simulink library "WECSim_Lib"  (R2015b)
settings: Solver=ode45  StartTime=0.0  StopTime=10.0  RelTol=1e-3
undefined symbols (not defined in the file): body, constraint, mooring, pto, simu, waves, X, Y, Z
libraries: nesl_utility x168, sm_lib x94, vrlib x12
(part 6 of 7)

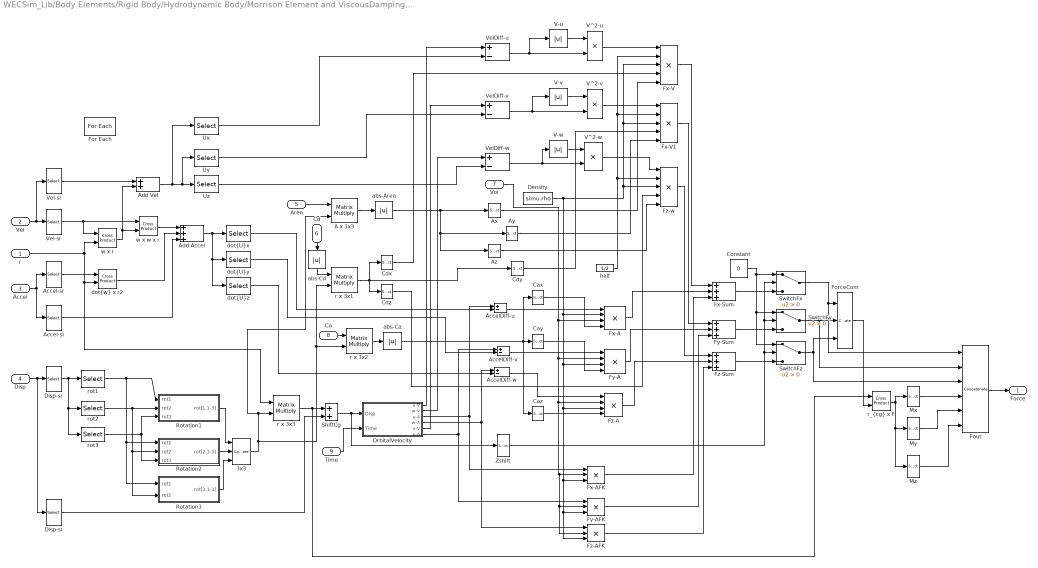
== system WECSim_Lib/Body Elements/Rigid Body/Hydrodynamic Body/Morrison Element and ViscousDampingForceCalculation/Morrison Element Variant Subsystem/Morrison Element On/No Wave Excitation Force/MorrisonElements ==
  r : Inport  Partition=on  PartitionDimension=1  PartitionWidth=1
  Vel : Inport  Port=2
  Accel : Inport  Port=3
  Disp : Inport  Port=4
  Area : Inport  Port=5  Partition=on  PartitionDimension=1  PartitionWidth=1
  Cd : Inport  Port=6  Partition=on  PartitionDimension=1  PartitionWidth=1
  Vol : Inport  Port=7  Partition=on  PartitionDimension=1  PartitionWidth=1
  Ca : Inport  Port=8  Partition=on  PartitionDimension=1  PartitionWidth=1
  Time : Inport  Port=9
  3x3 : Concatenate  NumInputs=3  Mode=Multidimensional array
  A x 3x3 : Product  Multiplication=Matrix(*)
  Accel-sl : Selector  InputPortWidth=6  IndexOptions=Index vector (dialog)  Indices=[1 2 3]  OutputSizes=1
  Accel-sr : Selector  InputPortWidth=6  IndexOptions=Index vector (dialog)  Indices=[4 5 6]  OutputSizes=1
  AccelDiff-u : Sum  Inputs=+-
  AccelDiff-v : Sum  Inputs=+-
  AccelDiff-w : Sum  Inputs=+-
  Add Accel : Sum  Inputs=+++
  Add Vel : Sum
  Ax : Selector  InputPortWidth=3  IndexOptions=Index vector (dialog)  Indices=[1]  OutputSizes=1
  Ay : Selector  InputPortWidth=3  IndexOptions=Index vector (dialog)  Indices=[2]  OutputSizes=1
  Az : Selector  InputPortWidth=3  IndexOptions=Index vector (dialog)  Indices=[3]  OutputSizes=1
  Cax : Selector  InputPortWidth=3  IndexOptions=Index vector (dialog)  Indices=[1]  OutputSizes=1
  Cay : Selector  InputPortWidth=3  IndexOptions=Index vector (dialog)  Indices=[2]  OutputSizes=1
  Caz : Selector  InputPortWidth=3  IndexOptions=Index vector (dialog)  Indices=[3]  OutputSizes=1
  Cdx : Selector  InputPortWidth=3  IndexOptions=Index vector (dialog)  Indices=[1]  OutputSizes=1
  Cdy : Selector  InputPortWidth=3  IndexOptions=Index vector (dialog)  Indices=[2]  OutputSizes=1
  Cdz : Selector  InputPortWidth=3  IndexOptions=Index vector (dialog)  Indices=[3]  OutputSizes=1
  Constant : Constant  Value=0
  Density : Constant  Value=simu.rho
  Disp-sl : Selector  InputPortWidth=6  IndexOptions=Index vector (dialog)  Indices=[1 2 3]  OutputSizes=1
  Disp-sr : Selector  InputPortWidth=6  IndexOptions=Index vector (dialog)  Indices=[4 5 6]  OutputSizes=1
  For Each : ForEach  DisableCoverage=on  IndexMode=One-based
  ForceCom : Concatenate  NumInputs=3  ConcatenateDimension=2
  Fout : Concatenate  NumInputs=6  Mode=Multidimensional array  ConcatenateDimension=2
  Fx-A : Product  Inputs=4
  Fx-AFK : Product  Inputs=3
  Fx-Sum : Sum  Inputs=+++
  Fx-V : Product  Inputs=5
  Fx-V1 : Product  Inputs=5
  Fy-A : Product  Inputs=4
  Fy-AFK : Product  Inputs=3
  Fy-Sum : Sum  Inputs=+++
  Fz-A : Product  Inputs=4
  Fz-AFK : Product  Inputs=3
  Fz-Sum : Sum  Inputs=+++
  Fz-w : Product  Inputs=5
  Mx : Selector  InputPortWidth=3  IndexOptions=Index vector (dialog)  Indices=[1]  OutputSizes=1
  My : Selector  InputPortWidth=3  IndexOptions=Index vector (dialog)  Indices=[2]  OutputSizes=1
  Mz : Selector  InputPortWidth=3  IndexOptions=Index vector (dialog)  Indices=[3]  OutputSizes=1
  OrbitalVelocity : Subsystem
  Rotation1 : Subsystem
  Rotation2 : Subsystem
  Rotation3 : Subsystem
  ShiftCg : Sum
  SwitchFx : Switch  Criteria=u2 > Threshold
  SwitchFy : Switch  Criteria=u2 > Threshold
  SwitchFz : Switch  Criteria=u2 > Threshold
  Ux : Selector  InputPortWidth=3  IndexOptions=Index vector (dialog)  Indices=[1]  OutputSizes=1
  Uy : Selector  InputPortWidth=3  IndexOptions=Index vector (dialog)  Indices=[2]  OutputSizes=1
  Uz : Selector  InputPortWidth=3  IndexOptions=Index vector (dialog)  Indices=[3]  OutputSizes=1
  V-u : Abs
  V-v : Abs
  V-w : Abs
  V^2-u : Product
  V^2-v : Product
  V^2-w : Product
  Vel-sl : Selector  InputPortWidth=6  IndexOptions=Index vector (dialog)  Indices=[1 2 3]  OutputSizes=1
  "Vel-sr " : Selector  InputPortWidth=6  IndexOptions=Index vector (dialog)  Indices=[4 5 6]  OutputSizes=1
  VelDiff-u : Sum  Inputs=+-
  VelDiff-v : Sum  Inputs=+-
  VelDiff-w : Sum  Inputs=+-
  Zshift : Selector  InputPortWidth=3  IndexOptions=Index vector (dialog)  Indices=[3]  OutputSizes=1
  abs-Area : Abs
  abs-Ca : Abs
  abs-Cd : Abs
  "dot{U}x" : Selector  InputPortWidth=3  IndexOptions=Index vector (dialog)  Indices=[1]  OutputSizes=1
  "dot{U}y" : Selector  InputPortWidth=3  IndexOptions=Index vector (dialog)  Indices=[2]  OutputSizes=1
  "dot{U}z" : Selector  InputPortWidth=3  IndexOptions=Index vector (dialog)  Indices=[3]  OutputSizes=1
  "dot{w} x r2" : vrlib/Utilities/Cross Product
  half : Constant  Value=1/2
  r x 3x1 : Product  Multiplication=Matrix(*)
  r x 3x2 : Product  Multiplication=Matrix(*)
  r x 3x3 : Product  Multiplication=Matrix(*)
  "r_{cg} x F" : vrlib/Utilities/Cross Product
  rot1 : Selector  InputPortWidth=3  IndexOptions=Index vector (dialog)  Indices=[1]  OutputSizes=1
  rot2 : Selector  InputPortWidth=3  IndexOptions=Index vector (dialog)  Indices=[2]  OutputSizes=1
  rot3 : Selector  InputPortWidth=3  IndexOptions=Index vector (dialog)  Indices=[3]  OutputSizes=1
  w x r : vrlib/Utilities/Cross Product
  w x w x r : vrlib/Utilities/Cross Product
  Force : Outport  PortDimensions=[1 6]  ConcatenationDimension=1
  wires:
  Vel/1 -> Vel-sl/1, "Vel-sr "/1
  w x r/1 -> Add Vel/2, w x w x r/2
  w x w x r/1 -> Add Accel/1
  "Vel-sr "/1 -> w x w x r/1, w x r/1
  r/1 -> r x 3x3/1, "dot{w} x r2"/2, w x r/2
  Accel/1 -> Accel-sl/1, Accel-sr/1
  Accel-sr/1 -> "dot{w} x r2"/1
  "dot{w} x r2"/1 -> Add Accel/2
  Accel-sl/1 -> Add Accel/3
  Add Accel/1 -> "dot{U}z"/1, "dot{U}y"/1, "dot{U}x"/1
  Vel-sl/1 -> Add Vel/1
  Disp/1 -> Disp-sl/1, Disp-sr/1
  Disp-sr/1 -> rot3/1, rot2/1, rot1/1
  rot3/1 -> Rotation2/3(rot3), Rotation1/3(rot3)
  rot1/1 -> Rotation3/1(rot1), Rotation2/1(rot1), Rotation1/1(rot1)
  rot2/1 -> Rotation3/2(rot2), Rotation2/2(rot2), Rotation1/2(rot2)
  Rotation2/1(rot[2,1-3]) -> 3x3/2
  Rotation1/1(rot[1,1-3]) -> 3x3/1
  Rotation3/1(rot[3,1-3]) -> 3x3/3
  r x 3x3/1 -> "r_{cg} x F"/1, ShiftCg/1
  Disp-sl/1 -> ShiftCg/2
  ShiftCg/1 -> Zshift/1, OrbitalVelocity/1(Disp)
  "dot{U}y"/1 -> AccelDiff-v/2
  "dot{U}x"/1 -> AccelDiff-u/2
  OrbitalVelocity/3(u-A) -> AccelDiff-u/1, Fx-AFK/1
  "dot{U}z"/1 -> AccelDiff-w/2
  Add Vel/1 -> Uy/1, Uz/1, Ux/1
  Uy/1 -> VelDiff-v/2
  Ux/1 -> VelDiff-u/2
  Uz/1 -> VelDiff-w/2
  OrbitalVelocity/1(u-V) -> VelDiff-u/1
  OrbitalVelocity/2(w-V) -> VelDiff-w/1
  VelDiff-w/1 -> V-w/1, V^2-w/2
  V^2-u/1 -> Fx-V/1
  half/1 -> Fz-w/2, Fx-V1/2, Fx-V/2
  Density/1 -> Fy-A/3, Fy-AFK/3, Fz-AFK/3, Fx-AFK/3, Fz-A/3, Fx-A/2, Fz-w/3, Fx-V1/3, Fx-V/3
  V^2-w/1 -> Fz-w/1
  AccelDiff-u/1 -> Fx-A/1
  Vol/1 -> Fy-A/2, Fy-AFK/2, Fz-AFK/2, Fx-AFK/2, Fz-A/2, Fx-A/3
  AccelDiff-w/1 -> Fz-A/1
  OrbitalVelocity/4(w-A) -> Fz-AFK/1, AccelDiff-w/1
  Fx-V/1 -> Fx-Sum/1
  Fx-A/1 -> Fx-Sum/2
  Fx-AFK/1 -> Fx-Sum/3
  Fz-w/1 -> Fz-Sum/1
  Fz-A/1 -> Fz-Sum/2
  Fz-AFK/1 -> Fz-Sum/3
  "r_{cg} x F"/1 -> Mz/1, My/1, Mx/1
  Mx/1 -> Fout/4
  My/1 -> Fout/5
  Mz/1 -> Fout/6
  3x3/1 -> A x 3x3/2, r x 3x3/2, r x 3x2/2, r x 3x1/2
  V-u/1 -> V^2-u/1
  VelDiff-u/1 -> V-u/1, V^2-u/2
  Zshift/1 -> SwitchFy/2, SwitchFx/2, SwitchFz/2
  SwitchFz/1 -> ForceCom/3, Fout/3
  SwitchFx/1 -> Fout/1, ForceCom/1
  Fx-Sum/1 -> SwitchFx/3
  Fz-Sum/1 -> SwitchFz/3
  Az/1 -> Fz-w/5
  Area/1 -> A x 3x3/1
  Ax/1 -> Fx-V/5
  Cdx/1 -> Fx-V/4
  Cdz/1 -> Fz-w/4
  A x 3x3/1 -> abs-Area/1
  abs-Area/1 -> Ay/1, Az/1, Ax/1
  ForceCom/1 -> "r_{cg} x F"/2
  Fout/1 -> Force/1
  Caz/1 -> Fz-A/4
  Cax/1 -> Fx-A/4
  Cd/1 -> abs-Cd/1
  r x 3x1/1 -> Cdy/1, Cdz/1, Cdx/1
  Ca/1 -> r x 3x2/1
  r x 3x2/1 -> abs-Ca/1
  OrbitalVelocity/6(v-A) -> AccelDiff-v/1, Fy-AFK/1
  V^2-v/1 -> Fx-V1/1
  V-v/1 -> V^2-v/1
  VelDiff-v/1 -> V-v/1, V^2-v/2
  OrbitalVelocity/5(v-V) -> VelDiff-v/1
  Ay/1 -> Fx-V1/5
  Cdy/1 -> Fx-V1/4
  SwitchFy/1 -> Fout/2, ForceCom/2
  Fy-Sum/1 -> SwitchFy/3
  Fy-AFK/1 -> Fy-Sum/3
  AccelDiff-v/1 -> Fy-A/1
  Cay/1 -> Fy-A/4
  Fy-A/1 -> Fy-Sum/2
  Fx-V1/1 -> Fy-Sum/1
  Constant/1 -> SwitchFy/1, SwitchFz/1, SwitchFx/1
  V-w/1 -> V^2-w/1
  abs-Ca/1 -> Cax/1, Cay/1, Caz/1
  abs-Cd/1 -> r x 3x1/1
  Time/1 -> OrbitalVelocity/2(Time)

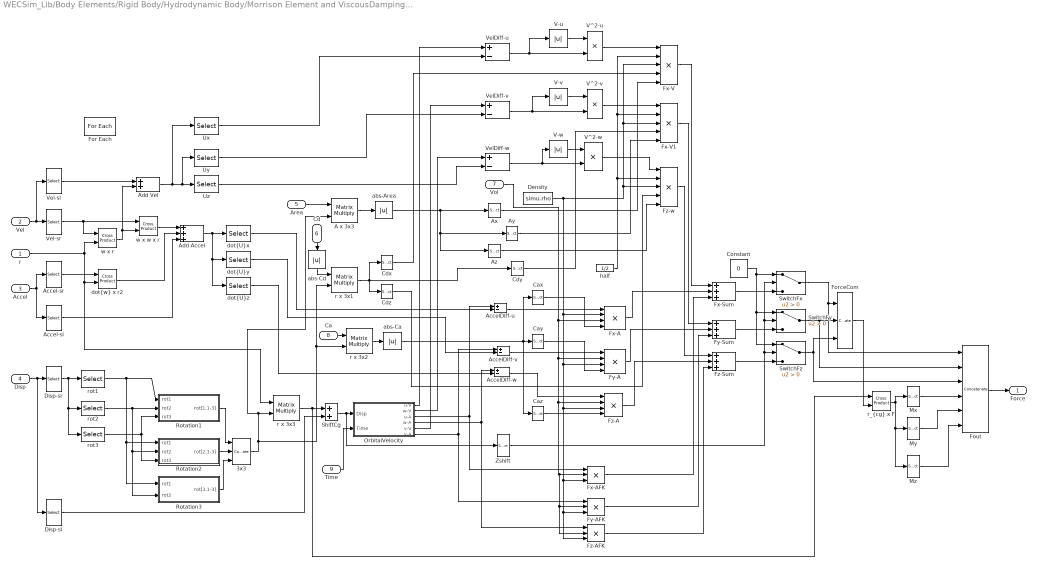
== system WECSim_Lib/Body Elements/Rigid Body/Hydrodynamic Body/Morrison Element and ViscousDampingForceCalculation/Morrison Element Variant Subsystem/Morrison Element On/Regular Wave Excitation Force/MorrisonElements ==
  r : Inport  Partition=on  PartitionDimension=1  PartitionWidth=1
  Vel : Inport  Port=2
  Accel : Inport  Port=3
  Disp : Inport  Port=4
  Area : Inport  Port=5  Partition=on  PartitionDimension=1  PartitionWidth=1
  Cd : Inport  Port=6  Partition=on  PartitionDimension=1  PartitionWidth=1
  Vol : Inport  Port=7  Partition=on  PartitionDimension=1  PartitionWidth=1
  Ca : Inport  Port=8  Partition=on  PartitionDimension=1  PartitionWidth=1
  Time : Inport  Port=9
  3x3 : Concatenate  NumInputs=3  Mode=Multidimensional array
  A x 3x3 : Product  Multiplication=Matrix(*)
  Accel-sl : Selector  InputPortWidth=6  IndexOptions=Index vector (dialog)  Indices=[1 2 3]  OutputSizes=1
  Accel-sr : Selector  InputPortWidth=6  IndexOptions=Index vector (dialog)  Indices=[4 5 6]  OutputSizes=1
  AccelDiff-u : Sum  Inputs=+-
  AccelDiff-v : Sum  Inputs=+-
  AccelDiff-w : Sum  Inputs=+-
  Add Accel : Sum  Inputs=+++
  Add Vel : Sum
  Ax : Selector  InputPortWidth=3  IndexOptions=Index vector (dialog)  Indices=[1]  OutputSizes=1
  Ay : Selector  InputPortWidth=3  IndexOptions=Index vector (dialog)  Indices=[2]  OutputSizes=1
  Az : Selector  InputPortWidth=3  IndexOptions=Index vector (dialog)  Indices=[3]  OutputSizes=1
  Cax : Selector  InputPortWidth=3  IndexOptions=Index vector (dialog)  Indices=[1]  OutputSizes=1
  Cay : Selector  InputPortWidth=3  IndexOptions=Index vector (dialog)  Indices=[2]  OutputSizes=1
  Caz : Selector  InputPortWidth=3  IndexOptions=Index vector (dialog)  Indices=[3]  OutputSizes=1
  Cdx : Selector  InputPortWidth=3  IndexOptions=Index vector (dialog)  Indices=[1]  OutputSizes=1
  Cdy : Selector  InputPortWidth=3  IndexOptions=Index vector (dialog)  Indices=[2]  OutputSizes=1
  Cdz : Selector  InputPortWidth=3  IndexOptions=Index vector (dialog)  Indices=[3]  OutputSizes=1
  Constant : Constant  Value=0
  Density : Constant  Value=simu.rho
  Disp-sl : Selector  InputPortWidth=6  IndexOptions=Index vector (dialog)  Indices=[1 2 3]  OutputSizes=1
  Disp-sr : Selector  InputPortWidth=6  IndexOptions=Index vector (dialog)  Indices=[4 5 6]  OutputSizes=1
  For Each : ForEach  DisableCoverage=on  IndexMode=One-based
  ForceCom : Concatenate  NumInputs=3  ConcatenateDimension=2
  Fout : Concatenate  NumInputs=6  Mode=Multidimensional array  ConcatenateDimension=2
  Fx-A : Product  Inputs=4
  Fx-AFK : Product  Inputs=3
  Fx-Sum : Sum  Inputs=+++
  Fx-V : Product  Inputs=5
  Fx-V1 : Product  Inputs=5
  Fy-A : Product  Inputs=4
  Fy-AFK : Product  Inputs=3
  Fy-Sum : Sum  Inputs=+++
  Fz-A : Product  Inputs=4
  Fz-AFK : Product  Inputs=3
  Fz-Sum : Sum  Inputs=+++
  Fz-w : Product  Inputs=5
  Mx : Selector  InputPortWidth=3  IndexOptions=Index vector (dialog)  Indices=[1]  OutputSizes=1
  My : Selector  InputPortWidth=3  IndexOptions=Index vector (dialog)  Indices=[2]  OutputSizes=1
  Mz : Selector  InputPortWidth=3  IndexOptions=Index vector (dialog)  Indices=[3]  OutputSizes=1
  OrbitalVelocity : Subsystem
  Rotation1 : Subsystem
  Rotation2 : Subsystem
  Rotation3 : Subsystem
  ShiftCg : Sum
  SwitchFx : Switch  Criteria=u2 > Threshold
  SwitchFy : Switch  Criteria=u2 > Threshold
  SwitchFz : Switch  Criteria=u2 > Threshold
  Ux : Selector  InputPortWidth=3  IndexOptions=Index vector (dialog)  Indices=[1]  OutputSizes=1
  Uy : Selector  InputPortWidth=3  IndexOptions=Index vector (dialog)  Indices=[2]  OutputSizes=1
  Uz : Selector  InputPortWidth=3  IndexOptions=Index vector (dialog)  Indices=[3]  OutputSizes=1
  V-u : Abs
  V-v : Abs
  V-w : Abs
  V^2-u : Product
  V^2-v : Product
  V^2-w : Product
  Vel-sl : Selector  InputPortWidth=6  IndexOptions=Index vector (dialog)  Indices=[1 2 3]  OutputSizes=1
  "Vel-sr " : Selector  InputPortWidth=6  IndexOptions=Index vector (dialog)  Indices=[4 5 6]  OutputSizes=1
  VelDiff-u : Sum  Inputs=+-
  VelDiff-v : Sum  Inputs=+-
  VelDiff-w : Sum  Inputs=+-
  Zshift : Selector  InputPortWidth=3  IndexOptions=Index vector (dialog)  Indices=[3]  OutputSizes=1
  abs-Area : Abs
  abs-Ca : Abs
  abs-Cd : Abs
  "dot{U}x" : Selector  InputPortWidth=3  IndexOptions=Index vector (dialog)  Indices=[1]  OutputSizes=1
  "dot{U}y" : Selector  InputPortWidth=3  IndexOptions=Index vector (dialog)  Indices=[2]  OutputSizes=1
  "dot{U}z" : Selector  InputPortWidth=3  IndexOptions=Index vector (dialog)  Indices=[3]  OutputSizes=1
  "dot{w} x r2" : vrlib/Utilities/Cross Product
  half : Constant  Value=1/2
  r x 3x1 : Product  Multiplication=Matrix(*)
  r x 3x2 : Product  Multiplication=Matrix(*)
  r x 3x3 : Product  Multiplication=Matrix(*)
  "r_{cg} x F" : vrlib/Utilities/Cross Product
  rot1 : Selector  InputPortWidth=3  IndexOptions=Index vector (dialog)  Indices=[1]  OutputSizes=1
  rot2 : Selector  InputPortWidth=3  IndexOptions=Index vector (dialog)  Indices=[2]  OutputSizes=1
  rot3 : Selector  InputPortWidth=3  IndexOptions=Index vector (dialog)  Indices=[3]  OutputSizes=1
  w x r : vrlib/Utilities/Cross Product
  w x w x r : vrlib/Utilities/Cross Product
  Force : Outport  PortDimensions=[1 6]  ConcatenationDimension=1
  wires:
  Vel/1 -> Vel-sl/1, "Vel-sr "/1
  w x r/1 -> Add Vel/2, w x w x r/2
  w x w x r/1 -> Add Accel/1
  "Vel-sr "/1 -> w x w x r/1, w x r/1
  r/1 -> r x 3x3/1, "dot{w} x r2"/2, w x r/2
  Accel/1 -> Accel-sl/1, Accel-sr/1
  Accel-sr/1 -> "dot{w} x r2"/1
  "dot{w} x r2"/1 -> Add Accel/2
  Accel-sl/1 -> Add Accel/3
  Add Accel/1 -> "dot{U}z"/1, "dot{U}y"/1, "dot{U}x"/1
  Vel-sl/1 -> Add Vel/1
  Disp/1 -> Disp-sl/1, Disp-sr/1
  Disp-sr/1 -> rot3/1, rot2/1, rot1/1
  rot3/1 -> Rotation2/3(rot3), Rotation1/3(rot3)
  rot1/1 -> Rotation3/1(rot1), Rotation2/1(rot1), Rotation1/1(rot1)
  rot2/1 -> Rotation3/2(rot2), Rotation2/2(rot2), Rotation1/2(rot2)
  Rotation2/1(rot[2,1-3]) -> 3x3/2
  Rotation1/1(rot[1,1-3]) -> 3x3/1
  Rotation3/1(rot[3,1-3]) -> 3x3/3
  r x 3x3/1 -> "r_{cg} x F"/1, ShiftCg/1
  Disp-sl/1 -> ShiftCg/2
  ShiftCg/1 -> Zshift/1, OrbitalVelocity/1(Disp)
  "dot{U}y"/1 -> AccelDiff-v/2
  "dot{U}x"/1 -> AccelDiff-u/2
  OrbitalVelocity/3(u-A) -> AccelDiff-u/1, Fx-AFK/1
  "dot{U}z"/1 -> AccelDiff-w/2
  Add Vel/1 -> Uy/1, Uz/1, Ux/1
  Uy/1 -> VelDiff-v/2
  Ux/1 -> VelDiff-u/2
  Uz/1 -> VelDiff-w/2
  OrbitalVelocity/1(u-V) -> VelDiff-u/1
  OrbitalVelocity/2(w-V) -> VelDiff-w/1
  VelDiff-w/1 -> V-w/1, V^2-w/2
  V^2-u/1 -> Fx-V/1
  half/1 -> Fz-w/2, Fx-V1/2, Fx-V/2
  Density/1 -> Fy-A/3, Fy-AFK/3, Fz-AFK/3, Fx-AFK/3, Fz-A/3, Fx-A/2, Fz-w/3, Fx-V1/3, Fx-V/3
  V^2-w/1 -> Fz-w/1
  AccelDiff-u/1 -> Fx-A/1
  Vol/1 -> Fy-A/2, Fy-AFK/2, Fz-AFK/2, Fx-AFK/2, Fz-A/2, Fx-A/3
  AccelDiff-w/1 -> Fz-A/1
  OrbitalVelocity/4(w-A) -> Fz-AFK/1, AccelDiff-w/1
  Fx-V/1 -> Fx-Sum/1
  Fx-A/1 -> Fx-Sum/2
  Fx-AFK/1 -> Fx-Sum/3
  Fz-w/1 -> Fz-Sum/1
  Fz-A/1 -> Fz-Sum/2
  Fz-AFK/1 -> Fz-Sum/3
  "r_{cg} x F"/1 -> Mz/1, My/1, Mx/1
  Mx/1 -> Fout/4
  My/1 -> Fout/5
  Mz/1 -> Fout/6
  3x3/1 -> A x 3x3/2, r x 3x3/2, r x 3x2/2, r x 3x1/2
  V-u/1 -> V^2-u/1
  VelDiff-u/1 -> V-u/1, V^2-u/2
  Zshift/1 -> SwitchFy/2, SwitchFx/2, SwitchFz/2
  SwitchFz/1 -> ForceCom/3, Fout/3
  SwitchFx/1 -> Fout/1, ForceCom/1
  Fx-Sum/1 -> SwitchFx/3
  Fz-Sum/1 -> SwitchFz/3
  Az/1 -> Fz-w/5
  Area/1 -> A x 3x3/1
  Ax/1 -> Fx-V/5
  Cdx/1 -> Fx-V/4
  Cdz/1 -> Fz-w/4
  A x 3x3/1 -> abs-Area/1
  abs-Area/1 -> Ay/1, Az/1, Ax/1
  ForceCom/1 -> "r_{cg} x F"/2
  Fout/1 -> Force/1
  Caz/1 -> Fz-A/4
  Cax/1 -> Fx-A/4
  Cd/1 -> abs-Cd/1
  r x 3x1/1 -> Cdy/1, Cdz/1, Cdx/1
  Ca/1 -> r x 3x2/1
  r x 3x2/1 -> abs-Ca/1
  OrbitalVelocity/6(v-A) -> AccelDiff-v/1, Fy-AFK/1
  V^2-v/1 -> Fx-V1/1
  V-v/1 -> V^2-v/1
  VelDiff-v/1 -> V-v/1, V^2-v/2
  OrbitalVelocity/5(v-V) -> VelDiff-v/1
  Ay/1 -> Fx-V1/5
  Cdy/1 -> Fx-V1/4
  SwitchFy/1 -> Fout/2, ForceCom/2
  Fy-Sum/1 -> SwitchFy/3
  Fy-AFK/1 -> Fy-Sum/3
  AccelDiff-v/1 -> Fy-A/1
  Cay/1 -> Fy-A/4
  Fy-A/1 -> Fy-Sum/2
  Fx-V1/1 -> Fy-Sum/1
  Constant/1 -> SwitchFy/1, SwitchFz/1, SwitchFx/1
  V-w/1 -> V^2-w/1
  abs-Ca/1 -> Cax/1, Cay/1, Caz/1
  abs-Cd/1 -> r x 3x1/1
  Time/1 -> OrbitalVelocity/2(Time)

== system WECSim_Lib/Body Elements/Rigid Body/Hydrodynamic Body/Morrison Element and ViscousDampingForceCalculation/Morrison Element Variant Subsystem/Morrison Element On/Irregular Wave Excitation Force/MorrisonElements/MorisonElementIrregular ==
  Disp : Inport
  waves.kirr : Inport  Port=2  Partition=on  PartitionDimension=1  PartitionWidth=1
  waves.w : Inport  Port=3  Partition=on  PartitionDimension=1  PartitionWidth=1
  waves.A : Inport  Port=4  Partition=on  PartitionDimension=1  PartitionWidth=1
  waves.RandPhase : Inport  Port=5  Partition=on  PartitionDimension=1  PartitionWidth=1
  Time : Inport  Port=6
  For Each : ForEach  DisableCoverage=on  IndexMode=One-based
  OrbitalVelocity : Subsystem
  u-V : Outport  ConcatenationDimension=1
  w-V : Outport  Port=2  ConcatenationDimension=1
  x-A : Outport  Port=3  ConcatenationDimension=1
  w-A : Outport  Port=4  ConcatenationDimension=1
  v-V : Outport  Port=5  ConcatenationDimension=1
  y-A : Outport  Port=6  ConcatenationDimension=1
  wires:
  Disp/1 -> OrbitalVelocity/1(Disp)
  waves.w/1 -> OrbitalVelocity/3(WaveFreq)
  waves.A/1 -> OrbitalVelocity/4(WaveAmp)
  waves.RandPhase/1 -> OrbitalVelocity/5(RandPhase)
  OrbitalVelocity/1(u-V) -> u-V/1
  OrbitalVelocity/2(w-V) -> w-V/1
  OrbitalVelocity/3(x-A) -> x-A/1
  OrbitalVelocity/4(w-A) -> w-A/1
  waves.kirr/1 -> OrbitalVelocity/2(WaveNumber)
  OrbitalVelocity/5(v-V) -> v-V/1
  OrbitalVelocity/6(y-A) -> y-A/1
  Time/1 -> OrbitalVelocity/6(Time)

== system WECSim_Lib/Body Elements/Rigid Body/Hydrodynamic Body/Morrison Element and ViscousDampingForceCalculation/Morrison Element Variant Subsystem/Morrison Element On/Irregular Wave Excitation Force/MorrisonElements/Rotation1 ==
  rot1 : Inport
  rot2 : Inport  Port=2
  rot3 : Inport  Port=3
  2 : Product
  3 : Product  Inputs=3
  7 : Product
  8 : Product  Inputs=3
  Combine : Concatenate  NumInputs=3  Mode=Multidimensional array  ConcatenateDimension=2
  Trigonometric Function{,1..2,6,9,11} (6 alike) : Trigonometry  Operator=cos
  Trigonometric Function{3..5,7..8,10} (6 alike) : Trigonometry
  rot11 : Product
  rot12 : Sum
  rot13 : Sum  Inputs=+-
  rot[1,1-3] : Outport
  wires:
  Trigonometric Function/1 -> rot11/1
  Trigonometric Function1/1 -> rot11/2
  rot11/1 -> Combine/1
  Trigonometric Function2/1 -> 2/1
  Trigonometric Function3/1 -> 2/2
  Trigonometric Function4/1 -> 3/1
  Trigonometric Function5/1 -> 3/2
  Trigonometric Function6/1 -> 3/3
  2/1 -> rot12/1
  3/1 -> rot12/2
  rot12/1 -> Combine/2
  Combine/1 -> rot[1,1-3]/1
  rot2/1 -> Trigonometric Function/1, Trigonometric Function5/1, Trigonometric Function10/1
  rot3/1 -> Trigonometric Function1/1, Trigonometric Function3/1, Trigonometric Function6/1, Trigonometric Function11/1, Trigonometric Function8/1
  rot1/1 -> Trigonometric Function2/1, Trigonometric Function4/1, Trigonometric Function9/1, Trigonometric Function7/1
  Trigonometric Function7/1 -> 7/1
  Trigonometric Function8/1 -> 7/2
  Trigonometric Function9/1 -> 8/1
  Trigonometric Function10/1 -> 8/2
  Trigonometric Function11/1 -> 8/3
  7/1 -> rot13/1
  8/1 -> rot13/2
  rot13/1 -> Combine/3

== system WECSim_Lib/Body Elements/Rigid Body/Hydrodynamic Body/Morrison Element and ViscousDampingForceCalculation/Morrison Element Variant Subsystem/Morrison Element On/Irregular Wave Excitation Force/MorrisonElements/Rotation2 ==
  rot1 : Inport
  rot2 : Inport  Port=2
  rot3 : Inport  Port=3
  2 : Product
  3 : Product  Inputs=3
  7 : Product
  8 : Product  Inputs=3
  Combine : Concatenate  NumInputs=3  Mode=Multidimensional array  ConcatenateDimension=2
  Gain : Gain  Gain=-1
  Trigonometric Function{,2..3,8..9} (5 alike) : Trigonometry  Operator=cos
  Trigonometric Function{1,4..7,10..11} (7 alike) : Trigonometry
  rot11 : Product
  rot12 : Sum  Inputs=+-
  rot13 : Sum
  rot[2,1-3] : Outport
  wires:
  Trigonometric Function/1 -> Gain/1
  Trigonometric Function1/1 -> rot11/2
  rot11/1 -> Combine/1
  Trigonometric Function2/1 -> 2/1
  Trigonometric Function3/1 -> 2/2
  Trigonometric Function4/1 -> 3/1
  Trigonometric Function5/1 -> 3/2
  Trigonometric Function6/1 -> 3/3
  2/1 -> rot12/1
  3/1 -> rot12/2
  rot12/1 -> Combine/2
  Combine/1 -> rot[2,1-3]/1
  rot2/1 -> Trigonometric Function/1, Trigonometric Function5/1, Trigonometric Function10/1
  rot3/1 -> Trigonometric Function1/1, Trigonometric Function3/1, Trigonometric Function6/1, Trigonometric Function11/1, Trigonometric Function8/1
  rot1/1 -> Trigonometric Function2/1, Trigonometric Function4/1, Trigonometric Function9/1, Trigonometric Function7/1
  Trigonometric Function7/1 -> 7/1
  Trigonometric Function8/1 -> 7/2
  Trigonometric Function9/1 -> 8/1
  Trigonometric Function10/1 -> 8/2
  Trigonometric Function11/1 -> 8/3
  7/1 -> rot13/1
  8/1 -> rot13/2
  rot13/1 -> Combine/3
  Gain/1 -> rot11/1

== system WECSim_Lib/Body Elements/Rigid Body/Hydrodynamic Body/Morrison Element and ViscousDampingForceCalculation/Morrison Element Variant Subsystem/Morrison Element On/Irregular Wave Excitation Force/MorrisonElements/Rotation3 ==
  rot1 : Inport
  rot2 : Inport  Port=2
  2 : Product
  7 : Product
  Combine : Concatenate  NumInputs=3  Mode=Multidimensional array  ConcatenateDimension=2
  Gain1 : Gain  Gain=-1
  TrigFun1 : Trigonometry
  TrigFun2 : Trigonometry
  TrigFun3 : Trigonometry  Operator=cos
  TrigFun4 : Trigonometry  Operator=cos
  TrigFun5 : Trigonometry  Operator=cos
  rot[3,1-3] : Outport
  wires:
  TrigFun1/1 -> Combine/1
  TrigFun3/1 -> 2/2
  2/1 -> Combine/2
  Combine/1 -> rot[3,1-3]/1
  rot2/1 -> TrigFun5/1, TrigFun3/1, TrigFun1/1
  TrigFun4/1 -> 7/1
  TrigFun5/1 -> 7/2
  rot1/1 -> TrigFun2/1, TrigFun4/1
  7/1 -> Combine/3
  TrigFun2/1 -> Gain1/1
  Gain1/1 -> 2/1

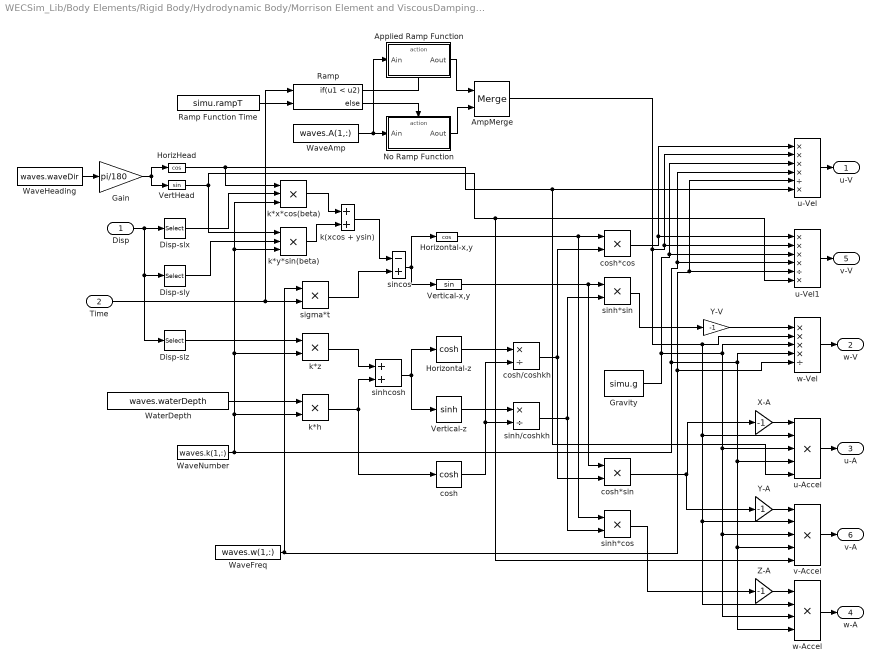
== system WECSim_Lib/Body Elements/Rigid Body/Hydrodynamic Body/Morrison Element and ViscousDampingForceCalculation/Morrison Element Variant Subsystem/Morrison Element On/No Wave Excitation Force/MorrisonElements/OrbitalVelocity ==
  Disp : Inport
  Time : Inport  Port=2
  AmpMerge : Merge
  Applied Ramp Function : Subsystem  TreatAsAtomicUnit=on
  Disp-slx : Selector  InputPortWidth=3  IndexOptions=Index vector (dialog)  Indices=[1]  OutputSizes=1
  Disp-sly : Selector  InputPortWidth=3  IndexOptions=Index vector (dialog)  Indices=[2]  OutputSizes=1
  Disp-slz : Selector  InputPortWidth=3  IndexOptions=Index vector (dialog)  Indices=[3]  OutputSizes=1
  Gain : Gain  Gain=pi/180
  Gravity : Constant  Value=simu.g
  HorizHead : Trigonometry  Operator=cos
  Horizontal-x,y : Trigonometry  Operator=cos
  Horizontal-z : Trigonometry  Operator=cosh
  No Ramp Function : Subsystem  TreatAsAtomicUnit=on
  Ramp : If  NumInputs=2  IfExpression=u1 < u2
  Ramp Function Time : Constant  Value=simu.rampT
  VertHead : Trigonometry
  Vertical-x,y : Trigonometry
  Vertical-z : Trigonometry  Operator=sinh
  WaterDepth : Constant  Value=waves.waterDepth
  WaveAmp : Constant  Value=waves.A(1,:)
  WaveFreq : Constant  Value=waves.w(1,:)
  WaveHeading : Constant  Value=waves.waveDir
  WaveNumber : Constant  Value=waves.k(1,:)
  X-A : Gain  Gain=-1
  Y-A : Gain  Gain=-1
  Y-V : Gain  Gain=-1
  Z-A : Gain  Gain=-1
  cosh : Trigonometry  Operator=cosh
  cosh*cos : Product  Inputs=**
  cosh*sin : Product  Inputs=**
  cosh/coshkh : Product  Inputs=*/
  k(xcos + ysin) : Sum
  k*h : Product
  k*x*cos(beta) : Product  Inputs=3
  k*y*sin(beta) : Product  Inputs=3
  k*z : Product
  sigma*t : Product
  sincos : Sum  Inputs=-+
  sinh*cos : Product  Inputs=**
  sinh*sin : Product  Inputs=**
  sinh/coshkh : Product  Inputs=*/
  sinhcosh : Sum
  u-Accel : Product  Inputs=*****
  u-Vel : Product  Inputs=****/*
  u-Vel1 : Product  Inputs=****/*
  v-Accel : Product  Inputs=*****
  w-Accel : Product  Inputs=****
  w-Vel : Product  Inputs=****/
  u-V : Outport
  w-V : Outport  Port=2
  u-A : Outport  Port=3
  w-A : Outport  Port=4
  v-V : Outport  Port=5
  v-A : Outport  Port=6
  wires:
  Disp/1 -> Disp-slz/1, Disp-sly/1, Disp-slx/1
  WaveNumber/1 -> k*h/2, k*z/2, k*y*sin(beta)/3, k*x*cos(beta)/3, w-Vel/4, v-Accel/4, w-Accel/4, u-Accel/4, u-Vel1/4, u-Vel/4
  WaterDepth/1 -> k*h/1
  sigma*t/1 -> sincos/2
  sincos/1 -> Vertical-x,y/1, Horizontal-x,y/1
  k*z/1 -> sinhcosh/1
  k*h/1 -> cosh/1, sinhcosh/2
  sinhcosh/1 -> Vertical-z/1, Horizontal-z/1
  Horizontal-z/1 -> cosh/coshkh/1
  cosh/1 -> sinh/coshkh/2, cosh/coshkh/2
  Vertical-z/1 -> sinh/coshkh/1
  Vertical-x,y/1 -> cosh*sin/1, sinh*sin/1
  sinh/coshkh/1 -> sinh*cos/2, sinh*sin/2
  Horizontal-x,y/1 -> sinh*cos/1, cosh*cos/1
  cosh/coshkh/1 -> cosh*cos/2, cosh*sin/2
  Disp-sly/1 -> k*y*sin(beta)/2
  cosh*cos/1 -> u-Vel1/1, u-Vel/1
  AmpMerge/1 -> w-Vel/2, w-Accel/2, v-Accel/2, u-Accel/2, u-Vel1/2, u-Vel/2
  Gravity/1 -> w-Vel/3, v-Accel/3, w-Accel/3, u-Accel/3, u-Vel1/3, u-Vel/3
  sinh*sin/1 -> Y-V/1
  Y-V/1 -> w-Vel/1
  X-A/1 -> u-Accel/1
  Z-A/1 -> w-Accel/1
  w-Vel/1 -> w-V/1
  u-Accel/1 -> u-A/1
  w-Accel/1 -> w-A/1
  cosh*sin/1 -> Y-A/1, X-A/1
  sinh*cos/1 -> Z-A/1
  Ramp Function Time/1 -> Ramp/2
  Ramp/2 -> No Ramp Function/Action
  Ramp/1 -> Applied Ramp Function/Action
  Time/1 -> Ramp/1, sigma*t/2
  No Ramp Function/1(Aout) -> AmpMerge/2
  Applied Ramp Function/1(Aout) -> AmpMerge/1
  Disp-slz/1 -> k*z/1
  WaveFreq/1 -> w-Vel/5, u-Vel1/5, u-Vel/5, sigma*t/1
  WaveAmp/1 -> Applied Ramp Function/1(Ain), No Ramp Function/1(Ain)
  WaveHeading/1 -> Gain/1
  Gain/1 -> HorizHead/1, VertHead/1
  Disp-slx/1 -> k*x*cos(beta)/2
  HorizHead/1 -> u-Accel/5, u-Vel/6, k*x*cos(beta)/1
  VertHead/1 -> k*y*sin(beta)/1, u-Vel1/6, v-Accel/5
  k*y*sin(beta)/1 -> k(xcos + ysin)/2
  k*x*cos(beta)/1 -> k(xcos + ysin)/1
  k(xcos + ysin)/1 -> sincos/1
  u-Vel1/1 -> v-V/1
  u-Vel/1 -> u-V/1
  Y-A/1 -> v-Accel/1
  v-Accel/1 -> v-A/1

== system WECSim_Lib/Body Elements/Rigid Body/Hydrodynamic Body/Morrison Element and ViscousDampingForceCalculation/Morrison Element Variant Subsystem/Morrison Element On/No Wave Excitation Force/MorrisonElements/Rotation1 ==
  rot1 : Inport
  rot2 : Inport  Port=2
  rot3 : Inport  Port=3
  2 : Product
  3 : Product  Inputs=3
  7 : Product
  8 : Product  Inputs=3
  Combine : Concatenate  NumInputs=3  Mode=Multidimensional array  ConcatenateDimension=2
  Trigonometric Function{,1..2,6,9,11} (6 alike) : Trigonometry  Operator=cos
  Trigonometric Function{3..5,7..8,10} (6 alike) : Trigonometry
  rot11 : Product
  rot12 : Sum
  rot13 : Sum  Inputs=+-
  rot[1,1-3] : Outport
  wires:
  Trigonometric Function/1 -> rot11/1
  Trigonometric Function1/1 -> rot11/2
  rot11/1 -> Combine/1
  Trigonometric Function2/1 -> 2/1
  Trigonometric Function3/1 -> 2/2
  Trigonometric Function4/1 -> 3/1
  Trigonometric Function5/1 -> 3/2
  Trigonometric Function6/1 -> 3/3
  2/1 -> rot12/1
  3/1 -> rot12/2
  rot12/1 -> Combine/2
  Combine/1 -> rot[1,1-3]/1
  rot2/1 -> Trigonometric Function/1, Trigonometric Function5/1, Trigonometric Function10/1
  rot3/1 -> Trigonometric Function1/1, Trigonometric Function3/1, Trigonometric Function6/1, Trigonometric Function11/1, Trigonometric Function8/1
  rot1/1 -> Trigonometric Function2/1, Trigonometric Function4/1, Trigonometric Function9/1, Trigonometric Function7/1
  Trigonometric Function7/1 -> 7/1
  Trigonometric Function8/1 -> 7/2
  Trigonometric Function9/1 -> 8/1
  Trigonometric Function10/1 -> 8/2
  Trigonometric Function11/1 -> 8/3
  7/1 -> rot13/1
  8/1 -> rot13/2
  rot13/1 -> Combine/3

== system WECSim_Lib/Body Elements/Rigid Body/Hydrodynamic Body/Morrison Element and ViscousDampingForceCalculation/Morrison Element Variant Subsystem/Morrison Element On/No Wave Excitation Force/MorrisonElements/Rotation2 ==
  rot1 : Inport
  rot2 : Inport  Port=2
  rot3 : Inport  Port=3
  2 : Product
  3 : Product  Inputs=3
  7 : Product
  8 : Product  Inputs=3
  Combine : Concatenate  NumInputs=3  Mode=Multidimensional array  ConcatenateDimension=2
  Gain : Gain  Gain=-1
  Trigonometric Function{,2..3,8..9} (5 alike) : Trigonometry  Operator=cos
  Trigonometric Function{1,4..7,10..11} (7 alike) : Trigonometry
  rot11 : Product
  rot12 : Sum  Inputs=+-
  rot13 : Sum
  rot[2,1-3] : Outport
  wires:
  Trigonometric Function/1 -> Gain/1
  Trigonometric Function1/1 -> rot11/2
  rot11/1 -> Combine/1
  Trigonometric Function2/1 -> 2/1
  Trigonometric Function3/1 -> 2/2
  Trigonometric Function4/1 -> 3/1
  Trigonometric Function5/1 -> 3/2
  Trigonometric Function6/1 -> 3/3
  2/1 -> rot12/1
  3/1 -> rot12/2
  rot12/1 -> Combine/2
  Combine/1 -> rot[2,1-3]/1
  rot2/1 -> Trigonometric Function/1, Trigonometric Function5/1, Trigonometric Function10/1
  rot3/1 -> Trigonometric Function1/1, Trigonometric Function3/1, Trigonometric Function6/1, Trigonometric Function11/1, Trigonometric Function8/1
  rot1/1 -> Trigonometric Function2/1, Trigonometric Function4/1, Trigonometric Function9/1, Trigonometric Function7/1
  Trigonometric Function7/1 -> 7/1
  Trigonometric Function8/1 -> 7/2
  Trigonometric Function9/1 -> 8/1
  Trigonometric Function10/1 -> 8/2
  Trigonometric Function11/1 -> 8/3
  7/1 -> rot13/1
  8/1 -> rot13/2
  rot13/1 -> Combine/3
  Gain/1 -> rot11/1

== system WECSim_Lib/Body Elements/Rigid Body/Hydrodynamic Body/Morrison Element and ViscousDampingForceCalculation/Morrison Element Variant Subsystem/Morrison Element On/No Wave Excitation Force/MorrisonElements/Rotation3 ==
  rot1 : Inport
  rot2 : Inport  Port=2
  2 : Product
  7 : Product
  Combine : Concatenate  NumInputs=3  Mode=Multidimensional array  ConcatenateDimension=2
  Gain1 : Gain  Gain=-1
  TrigFun1 : Trigonometry
  TrigFun2 : Trigonometry
  TrigFun3 : Trigonometry  Operator=cos
  TrigFun4 : Trigonometry  Operator=cos
  TrigFun5 : Trigonometry  Operator=cos
  rot[3,1-3] : Outport
  wires:
  TrigFun1/1 -> Combine/1
  TrigFun3/1 -> 2/2
  2/1 -> Combine/2
  Combine/1 -> rot[3,1-3]/1
  rot2/1 -> TrigFun5/1, TrigFun3/1, TrigFun1/1
  TrigFun4/1 -> 7/1
  TrigFun5/1 -> 7/2
  rot1/1 -> TrigFun2/1, TrigFun4/1
  7/1 -> Combine/3
  TrigFun2/1 -> Gain1/1
  Gain1/1 -> 2/1

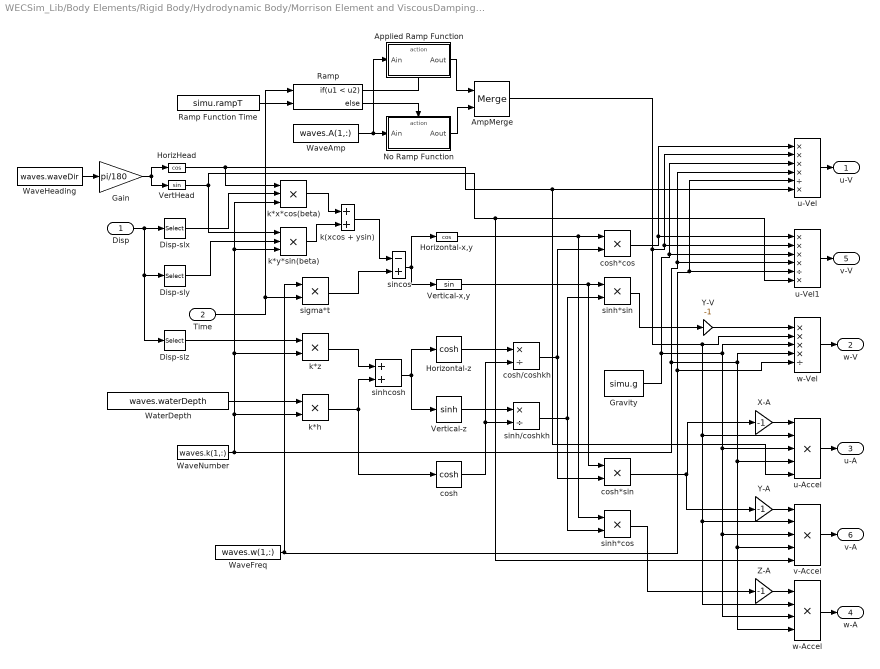
== system WECSim_Lib/Body Elements/Rigid Body/Hydrodynamic Body/Morrison Element and ViscousDampingForceCalculation/Morrison Element Variant Subsystem/Morrison Element On/Regular Wave Excitation Force/MorrisonElements/OrbitalVelocity ==
  Disp : Inport
  Time : Inport  Port=2
  AmpMerge : Merge
  Applied Ramp Function : Subsystem  TreatAsAtomicUnit=on
  Disp-slx : Selector  InputPortWidth=3  IndexOptions=Index vector (dialog)  Indices=[1]  OutputSizes=1
  Disp-sly : Selector  InputPortWidth=3  IndexOptions=Index vector (dialog)  Indices=[2]  OutputSizes=1
  Disp-slz : Selector  InputPortWidth=3  IndexOptions=Index vector (dialog)  Indices=[3]  OutputSizes=1
  Gain : Gain  Gain=pi/180
  Gravity : Constant  Value=simu.g
  HorizHead : Trigonometry  Operator=cos
  Horizontal-x,y : Trigonometry  Operator=cos
  Horizontal-z : Trigonometry  Operator=cosh
  No Ramp Function : Subsystem  TreatAsAtomicUnit=on
  Ramp : If  NumInputs=2  IfExpression=u1 < u2
  Ramp Function Time : Constant  Value=simu.rampT
  VertHead : Trigonometry
  Vertical-x,y : Trigonometry
  Vertical-z : Trigonometry  Operator=sinh
  WaterDepth : Constant  Value=waves.waterDepth
  WaveAmp : Constant  Value=waves.A(1,:)
  WaveFreq : Constant  Value=waves.w(1,:)
  WaveHeading : Constant  Value=waves.waveDir
  WaveNumber : Constant  Value=waves.k(1,:)
  X-A : Gain  Gain=-1
  Y-A : Gain  Gain=-1
  Y-V : Gain  Gain=-1
  Z-A : Gain  Gain=-1
  cosh : Trigonometry  Operator=cosh
  cosh*cos : Product  Inputs=**
  cosh*sin : Product  Inputs=**
  cosh/coshkh : Product  Inputs=*/
  k(xcos + ysin) : Sum
  k*h : Product
  k*x*cos(beta) : Product  Inputs=3
  k*y*sin(beta) : Product  Inputs=3
  k*z : Product
  sigma*t : Product
  sincos : Sum  Inputs=-+
  sinh*cos : Product  Inputs=**
  sinh*sin : Product  Inputs=**
  sinh/coshkh : Product  Inputs=*/
  sinhcosh : Sum
  u-Accel : Product  Inputs=*****
  u-Vel : Product  Inputs=****/*
  u-Vel1 : Product  Inputs=****/*
  v-Accel : Product  Inputs=*****
  w-Accel : Product  Inputs=****
  w-Vel : Product  Inputs=****/
  u-V : Outport
  w-V : Outport  Port=2
  u-A : Outport  Port=3
  w-A : Outport  Port=4
  v-V : Outport  Port=5
  v-A : Outport  Port=6
  wires:
  Disp/1 -> Disp-slz/1, Disp-sly/1, Disp-slx/1
  WaveNumber/1 -> k*h/2, k*z/2, k*y*sin(beta)/3, k*x*cos(beta)/3, w-Vel/4, v-Accel/4, w-Accel/4, u-Accel/4, u-Vel1/4, u-Vel/4
  WaterDepth/1 -> k*h/1
  sigma*t/1 -> sincos/2
  sincos/1 -> Vertical-x,y/1, Horizontal-x,y/1
  k*z/1 -> sinhcosh/1
  k*h/1 -> cosh/1, sinhcosh/2
  sinhcosh/1 -> Vertical-z/1, Horizontal-z/1
  Horizontal-z/1 -> cosh/coshkh/1
  cosh/1 -> sinh/coshkh/2, cosh/coshkh/2
  Vertical-z/1 -> sinh/coshkh/1
  Vertical-x,y/1 -> cosh*sin/1, sinh*sin/1
  sinh/coshkh/1 -> sinh*cos/2, sinh*sin/2
  Horizontal-x,y/1 -> sinh*cos/1, cosh*cos/1
  cosh/coshkh/1 -> cosh*cos/2, cosh*sin/2
  Disp-sly/1 -> k*y*sin(beta)/2
  cosh*cos/1 -> u-Vel1/1, u-Vel/1
  AmpMerge/1 -> w-Vel/2, w-Accel/2, v-Accel/2, u-Accel/2, u-Vel1/2, u-Vel/2
  Gravity/1 -> w-Vel/3, v-Accel/3, w-Accel/3, u-Accel/3, u-Vel1/3, u-Vel/3
  sinh*sin/1 -> Y-V/1
  Y-V/1 -> w-Vel/1
  X-A/1 -> u-Accel/1
  Z-A/1 -> w-Accel/1
  w-Vel/1 -> w-V/1
  u-Accel/1 -> u-A/1
  w-Accel/1 -> w-A/1
  cosh*sin/1 -> Y-A/1, X-A/1
  sinh*cos/1 -> Z-A/1
  Ramp Function Time/1 -> Ramp/2
  Ramp/2 -> No Ramp Function/Action
  Ramp/1 -> Applied Ramp Function/Action
  Time/1 -> Ramp/1, sigma*t/2
  No Ramp Function/1(Aout) -> AmpMerge/2
  Applied Ramp Function/1(Aout) -> AmpMerge/1
  Disp-slz/1 -> k*z/1
  WaveFreq/1 -> w-Vel/5, u-Vel1/5, u-Vel/5, sigma*t/1
  WaveAmp/1 -> Applied Ramp Function/1(Ain), No Ramp Function/1(Ain)
  WaveHeading/1 -> Gain/1
  Gain/1 -> HorizHead/1, VertHead/1
  Disp-slx/1 -> k*x*cos(beta)/2
  HorizHead/1 -> u-Accel/5, u-Vel/6, k*x*cos(beta)/1
  VertHead/1 -> k*y*sin(beta)/1, u-Vel1/6, v-Accel/5
  k*y*sin(beta)/1 -> k(xcos + ysin)/2
  k*x*cos(beta)/1 -> k(xcos + ysin)/1
  k(xcos + ysin)/1 -> sincos/1
  u-Vel1/1 -> v-V/1
  u-Vel/1 -> u-V/1
  Y-A/1 -> v-Accel/1
  v-Accel/1 -> v-A/1

== system WECSim_Lib/Body Elements/Rigid Body/Hydrodynamic Body/Morrison Element and ViscousDampingForceCalculation/Morrison Element Variant Subsystem/Morrison Element On/Regular Wave Excitation Force/MorrisonElements/Rotation1 ==
  rot1 : Inport
  rot2 : Inport  Port=2
  rot3 : Inport  Port=3
  2 : Product
  3 : Product  Inputs=3
  7 : Product
  8 : Product  Inputs=3
  Combine : Concatenate  NumInputs=3  Mode=Multidimensional array  ConcatenateDimension=2
  Trigonometric Function{,1..2,6,9,11} (6 alike) : Trigonometry  Operator=cos
  Trigonometric Function{3..5,7..8,10} (6 alike) : Trigonometry
  rot11 : Product
  rot12 : Sum
  rot13 : Sum  Inputs=+-
  rot[1,1-3] : Outport
  wires:
  Trigonometric Function/1 -> rot11/1
  Trigonometric Function1/1 -> rot11/2
  rot11/1 -> Combine/1
  Trigonometric Function2/1 -> 2/1
  Trigonometric Function3/1 -> 2/2
  Trigonometric Function4/1 -> 3/1
  Trigonometric Function5/1 -> 3/2
  Trigonometric Function6/1 -> 3/3
  2/1 -> rot12/1
  3/1 -> rot12/2
  rot12/1 -> Combine/2
  Combine/1 -> rot[1,1-3]/1
  rot2/1 -> Trigonometric Function/1, Trigonometric Function5/1, Trigonometric Function10/1
  rot3/1 -> Trigonometric Function1/1, Trigonometric Function3/1, Trigonometric Function6/1, Trigonometric Function11/1, Trigonometric Function8/1
  rot1/1 -> Trigonometric Function2/1, Trigonometric Function4/1, Trigonometric Function9/1, Trigonometric Function7/1
  Trigonometric Function7/1 -> 7/1
  Trigonometric Function8/1 -> 7/2
  Trigonometric Function9/1 -> 8/1
  Trigonometric Function10/1 -> 8/2
  Trigonometric Function11/1 -> 8/3
  7/1 -> rot13/1
  8/1 -> rot13/2
  rot13/1 -> Combine/3

== system WECSim_Lib/Body Elements/Rigid Body/Hydrodynamic Body/Morrison Element and ViscousDampingForceCalculation/Morrison Element Variant Subsystem/Morrison Element On/Regular Wave Excitation Force/MorrisonElements/Rotation2 ==
  rot1 : Inport
  rot2 : Inport  Port=2
  rot3 : Inport  Port=3
  2 : Product
  3 : Product  Inputs=3
  7 : Product
  8 : Product  Inputs=3
  Combine : Concatenate  NumInputs=3  Mode=Multidimensional array  ConcatenateDimension=2
  Gain : Gain  Gain=-1
  Trigonometric Function{,2..3,8..9} (5 alike) : Trigonometry  Operator=cos
  Trigonometric Function{1,4..7,10..11} (7 alike) : Trigonometry
  rot11 : Product
  rot12 : Sum  Inputs=+-
  rot13 : Sum
  rot[2,1-3] : Outport
  wires:
  Trigonometric Function/1 -> Gain/1
  Trigonometric Function1/1 -> rot11/2
  rot11/1 -> Combine/1
  Trigonometric Function2/1 -> 2/1
  Trigonometric Function3/1 -> 2/2
  Trigonometric Function4/1 -> 3/1
  Trigonometric Function5/1 -> 3/2
  Trigonometric Function6/1 -> 3/3
  2/1 -> rot12/1
  3/1 -> rot12/2
  rot12/1 -> Combine/2
  Combine/1 -> rot[2,1-3]/1
  rot2/1 -> Trigonometric Function/1, Trigonometric Function5/1, Trigonometric Function10/1
  rot3/1 -> Trigonometric Function1/1, Trigonometric Function3/1, Trigonometric Function6/1, Trigonometric Function11/1, Trigonometric Function8/1
  rot1/1 -> Trigonometric Function2/1, Trigonometric Function4/1, Trigonometric Function9/1, Trigonometric Function7/1
  Trigonometric Function7/1 -> 7/1
  Trigonometric Function8/1 -> 7/2
  Trigonometric Function9/1 -> 8/1
  Trigonometric Function10/1 -> 8/2
  Trigonometric Function11/1 -> 8/3
  7/1 -> rot13/1
  8/1 -> rot13/2
  rot13/1 -> Combine/3
  Gain/1 -> rot11/1

== system WECSim_Lib/Body Elements/Rigid Body/Hydrodynamic Body/Morrison Element and ViscousDampingForceCalculation/Morrison Element Variant Subsystem/Morrison Element On/Regular Wave Excitation Force/MorrisonElements/Rotation3 ==
  rot1 : Inport
  rot2 : Inport  Port=2
  2 : Product
  7 : Product
  Combine : Concatenate  NumInputs=3  Mode=Multidimensional array  ConcatenateDimension=2
  Gain1 : Gain  Gain=-1
  TrigFun1 : Trigonometry
  TrigFun2 : Trigonometry
  TrigFun3 : Trigonometry  Operator=cos
  TrigFun4 : Trigonometry  Operator=cos
  TrigFun5 : Trigonometry  Operator=cos
  rot[3,1-3] : Outport
  wires:
  TrigFun1/1 -> Combine/1
  TrigFun3/1 -> 2/2
  2/1 -> Combine/2
  Combine/1 -> rot[3,1-3]/1
  rot2/1 -> TrigFun5/1, TrigFun3/1, TrigFun1/1
  TrigFun4/1 -> 7/1
  TrigFun5/1 -> 7/2
  rot1/1 -> TrigFun2/1, TrigFun4/1
  7/1 -> Combine/3
  TrigFun2/1 -> Gain1/1
  Gain1/1 -> 2/1

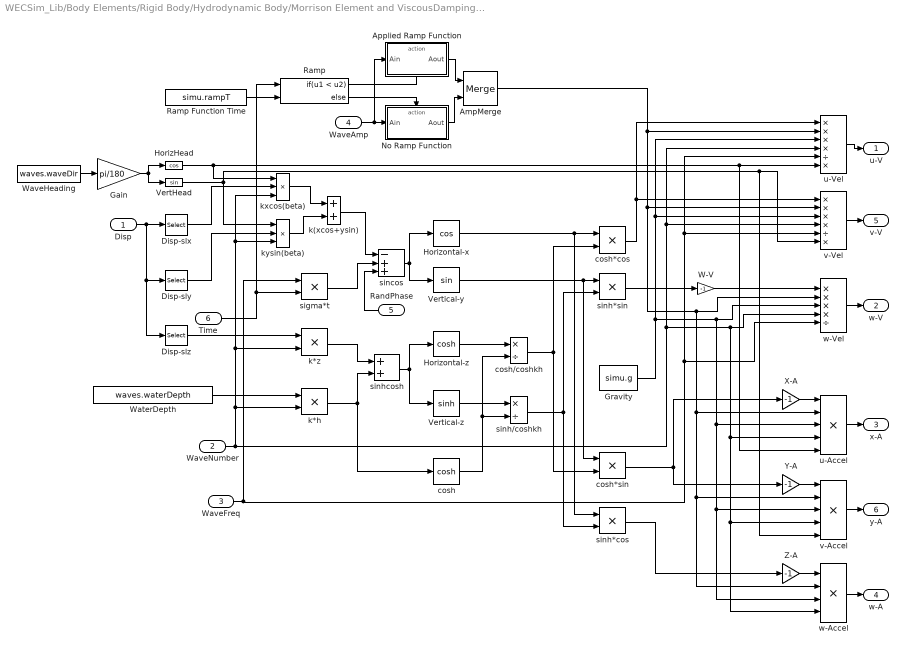
== system WECSim_Lib/Body Elements/Rigid Body/Hydrodynamic Body/Morrison Element and ViscousDampingForceCalculation/Morrison Element Variant Subsystem/Morrison Element On/Irregular Wave Excitation Force/MorrisonElements/MorisonElementIrregular/OrbitalVelocity ==
  Disp : Inport
  WaveNumber : Inport  Port=2
  WaveFreq : Inport  Port=3
  WaveAmp : Inport  Port=4
  RandPhase : Inport  Port=5
  Time : Inport  Port=6
  AmpMerge : Merge
  Applied Ramp Function : Subsystem  TreatAsAtomicUnit=on
  Disp-slx : Selector  InputPortWidth=3  IndexOptions=Index vector (dialog)  Indices=[1]  OutputSizes=1
  Disp-sly : Selector  InputPortWidth=3  IndexOptions=Index vector (dialog)  Indices=[2]  OutputSizes=1
  Disp-slz : Selector  InputPortWidth=3  IndexOptions=Index vector (dialog)  Indices=[3]  OutputSizes=1
  Gain : Gain  Gain=pi/180
  Gravity : Constant  Value=simu.g
  HorizHead : Trigonometry  Operator=cos
  Horizontal-x : Trigonometry  Operator=cos
  Horizontal-z : Trigonometry  Operator=cosh
  No Ramp Function : Subsystem  TreatAsAtomicUnit=on
  Ramp : If  NumInputs=2  IfExpression=u1 < u2
  Ramp Function Time : Constant  Value=simu.rampT
  VertHead : Trigonometry
  Vertical-y : Trigonometry
  Vertical-z : Trigonometry  Operator=sinh
  W-V : Gain  Gain=-1
  WaterDepth : Constant  Value=waves.waterDepth
  WaveHeading : Constant  Value=waves.waveDir
  X-A : Gain  Gain=-1
  Y-A : Gain  Gain=-1
  Z-A : Gain  Gain=-1
  cosh : Trigonometry  Operator=cosh
  cosh*cos : Product  Inputs=**
  cosh*sin : Product  Inputs=**
  cosh/coshkh : Product  Inputs=*/
  k(xcos+ysin) : Sum
  k*h : Product
  k*z : Product
  kxcos(beta) : Product  Inputs=3
  kysin(beta) : Product  Inputs=3
  sigma*t : Product
  sincos : Sum  Inputs=-++
  sinh*cos : Product  Inputs=**
  sinh*sin : Product  Inputs=**
  sinh/coshkh : Product  Inputs=*/
  sinhcosh : Sum
  u-Accel : Product  Inputs=*****
  u-Vel : Product  Inputs=****/*
  v-Accel : Product  Inputs=*****
  v-Vel : Product  Inputs=****/*
  w-Accel : Product  Inputs=****
  w-Vel : Product  Inputs=****/
  u-V : Outport
  w-V : Outport  Port=2
  x-A : Outport  Port=3
  w-A : Outport  Port=4
  v-V : Outport  Port=5
  y-A : Outport  Port=6
  wires:
  Disp/1 -> Disp-slz/1, Disp-sly/1, Disp-slx/1
  WaveNumber/1 -> w-Vel/4, v-Accel/4, w-Accel/4, u-Accel/4, u-Vel/4, v-Vel/4, k*h/2, k*z/2, kysin(beta)/3, kxcos(beta)/3
  WaveFreq/1 -> sigma*t/1, u-Vel/5, v-Vel/5, w-Vel/5
  WaterDepth/1 -> k*h/1
  sigma*t/1 -> sincos/2
  sincos/1 -> Vertical-y/1, Horizontal-x/1
  k*z/1 -> sinhcosh/1
  k*h/1 -> cosh/1, sinhcosh/2
  sinhcosh/1 -> Vertical-z/1, Horizontal-z/1
  Horizontal-z/1 -> cosh/coshkh/1
  cosh/1 -> sinh/coshkh/2, cosh/coshkh/2
  Vertical-z/1 -> sinh/coshkh/1
  Vertical-y/1 -> sinh*sin/1, cosh*sin/1
  sinh/coshkh/1 -> sinh*cos/2, sinh*sin/2
  Horizontal-x/1 -> cosh*cos/1, sinh*cos/1
  cosh/coshkh/1 -> cosh*cos/2, cosh*sin/2
  Disp-sly/1 -> kysin(beta)/2
  cosh*cos/1 -> u-Vel/1, v-Vel/1
  AmpMerge/1 -> w-Vel/2, w-Accel/2, v-Accel/2, u-Accel/2, v-Vel/2, u-Vel/2
  sinh*sin/1 -> W-V/1
  W-V/1 -> w-Vel/1
  X-A/1 -> u-Accel/1
  Z-A/1 -> w-Accel/1
  u-Vel/1 -> u-V/1
  w-Vel/1 -> w-V/1
  u-Accel/1 -> x-A/1
  w-Accel/1 -> w-A/1
  cosh*sin/1 -> Y-A/1, X-A/1
  sinh*cos/1 -> Z-A/1
  Ramp Function Time/1 -> Ramp/2
  Ramp/2 -> No Ramp Function/Action
  Ramp/1 -> Applied Ramp Function/Action
  Time/1 -> sigma*t/2, Ramp/1
  WaveAmp/1 -> Applied Ramp Function/1(Ain), No Ramp Function/1(Ain)
  No Ramp Function/1(Aout) -> AmpMerge/2
  Applied Ramp Function/1(Aout) -> AmpMerge/1
  Disp-slz/1 -> k*z/1
  RandPhase/1 -> sincos/3
  WaveHeading/1 -> Gain/1
  Gain/1 -> HorizHead/1, VertHead/1
  Disp-slx/1 -> kxcos(beta)/2
  HorizHead/1 -> kxcos(beta)/1, u-Vel/6, u-Accel/5
  VertHead/1 -> kysin(beta)/1, v-Accel/5, v-Vel/6
  kysin(beta)/1 -> k(xcos+ysin)/2
  kxcos(beta)/1 -> k(xcos+ysin)/1
  k(xcos+ysin)/1 -> sincos/1
  v-Vel/1 -> v-V/1
  Gravity/1 -> w-Vel/3, v-Accel/3, w-Accel/3, u-Accel/3, u-Vel/3, v-Vel/3
  Y-A/1 -> v-Accel/1
  v-Accel/1 -> y-A/1

== system WECSim_Lib/Body Elements/Rigid Body/Hydrodynamic Body/Morrison Element and ViscousDampingForceCalculation/Morrison Element Variant Subsystem/Morrison Element On/No Wave Excitation Force/MorrisonElements/OrbitalVelocity/Applied Ramp Function ==
  Ain : Inport
  Action Port : ActionPort
  Add : Sum
  Constant : Constant  Value=2
  Constant1 : Constant
  Divide : Product  Inputs=**/
  Sine Wave : Sin  Frequency=pi/simu.rampT  Phase=pi+pi/2  SampleTime=0
  Aout : Outport
  wires:
  Ain/1 -> Divide/1
  Divide/1 -> Aout/1
  Constant/1 -> Divide/3
  Constant1/1 -> Add/1
  Sine Wave/1 -> Add/2
  Add/1 -> Divide/2

== system WECSim_Lib/Body Elements/Rigid Body/Hydrodynamic Body/Morrison Element and ViscousDampingForceCalculation/Morrison Element Variant Subsystem/Morrison Element On/No Wave Excitation Force/MorrisonElements/OrbitalVelocity/No Ramp Function ==
  Ain : Inport
  Action Port : ActionPort
  Aout : Outport
  wires:
  Ain/1 -> Aout/1

== system WECSim_Lib/Body Elements/Rigid Body/Hydrodynamic Body/Morrison Element and ViscousDampingForceCalculation/Morrison Element Variant Subsystem/Morrison Element On/Regular Wave Excitation Force/MorrisonElements/OrbitalVelocity/Applied Ramp Function ==
  Ain : Inport
  Action Port : ActionPort
  Add : Sum
  Constant : Constant  Value=2
  Constant1 : Constant
  Divide : Product  Inputs=**/
  Sine Wave : Sin  Frequency=pi/simu.rampT  Phase=pi+pi/2  SampleTime=0
  Aout : Outport
  wires:
  Ain/1 -> Divide/1
  Divide/1 -> Aout/1
  Constant/1 -> Divide/3
  Constant1/1 -> Add/1
  Sine Wave/1 -> Add/2
  Add/1 -> Divide/2

== system WECSim_Lib/Body Elements/Rigid Body/Hydrodynamic Body/Morrison Element and ViscousDampingForceCalculation/Morrison Element Variant Subsystem/Morrison Element On/Regular Wave Excitation Force/MorrisonElements/OrbitalVelocity/No Ramp Function ==
  Ain : Inport
  Action Port : ActionPort
  Aout : Outport
  wires:
  Ain/1 -> Aout/1

== system WECSim_Lib/Body Elements/Rigid Body/Hydrodynamic Body/Morrison Element and ViscousDampingForceCalculation/Morrison Element Variant Subsystem/Morrison Element On/Irregular Wave Excitation Force/MorrisonElements/MorisonElementIrregular/OrbitalVelocity/Applied Ramp Function ==
  Ain : Inport
  Action Port : ActionPort
  Add : Sum
  Constant : Constant  Value=2
  Constant1 : Constant
  Divide : Product  Inputs=**/
  Sine Wave : Sin  Frequency=pi/simu.rampT  Phase=pi+pi/2  SampleTime=0
  Aout : Outport
  wires:
  Ain/1 -> Divide/1
  Divide/1 -> Aout/1
  Constant/1 -> Divide/3
  Constant1/1 -> Add/1
  Sine Wave/1 -> Add/2
  Add/1 -> Divide/2

== system WECSim_Lib/Body Elements/Rigid Body/Hydrodynamic Body/Morrison Element and ViscousDampingForceCalculation/Morrison Element Variant Subsystem/Morrison Element On/Irregular Wave Excitation Force/MorrisonElements/MorisonElementIrregular/OrbitalVelocity/No Ramp Function ==
  Ain : Inport
  Action Port : ActionPort
  Aout : Outport
  wires:
  Ain/1 -> Aout/1
